simulink model "prob6"  (R2020b)
settings: Solver=VariableStepAuto  StartTime=0.0  StopTime=10.0  RelTol=1e-3
settings Model: Creator=Admin  LastModifiedBy=Admin

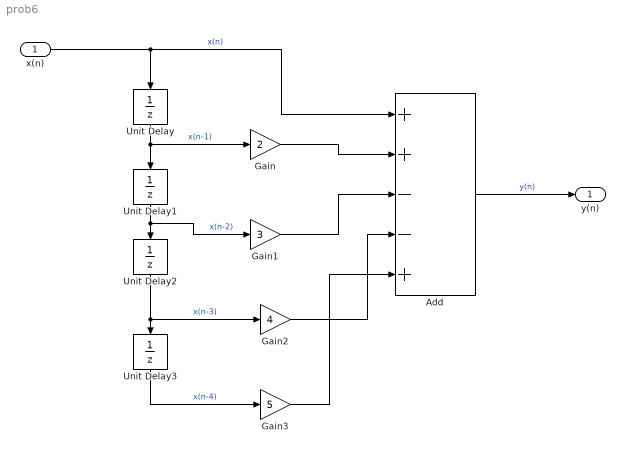
== system prob6 ==
  x(n) : Inport
  Add : Sum  Inputs=++--+
  Gain : Gain  Gain=2
  Gain1 : Gain  Gain=3
  Gain2 : Gain  Gain=4
  Gain3 : Gain  Gain=5
  Unit Delay{,1..3} (4 alike) : UnitDelay  SampleTime=-1  HasFrameUpgradeWarning=on
  y(n) : Outport
  wires:
  Unit Delay/1 -> Gain/1, Unit Delay1/1  "x(n-1)"
  Unit Delay1/1 -> Gain1/1, Unit Delay2/1  "x(n-2)"
  Unit Delay2/1 -> Gain2/1, Unit Delay3/1  "x(n-3)"
  Unit Delay3/1 -> Gain3/1  "x(n-4)"
  x(n)/1 -> Unit Delay/1, Add/1  "x(n)"
  Gain/1 -> Add/2
  Gain1/1 -> Add/3
  Gain2/1 -> Add/4
  Gain3/1 -> Add/5
  Add/1 -> y(n)/1  "y(n)"
